simulink model "casihi"  (R2022b)
settings: Solver=VariableStepAuto  StartTime=0.0  StopTime=50  RelTol=1e-3
settings Model: Creator=10911  LastModifiedBy=acer
settings SolverCC: AlgebraicLoopSolver=TrustRegion
settings OptimizationCC: LifeSpan=inf
settings DebuggingCC: UnconnectedInputMsg=warning  UnconnectedOutputMsg=warning  UnconnectedLineMsg=warning  SFMachineParentedDataDiag=warning  ArithmeticOperatorsInVariantConditions=warning
settings ModelReferenceCC: EnableRefExpFcnMdlSchedulingChecks=on
settings SFSimCC: CustomCodeUndefinedFunction=UseInterfaceOnly
settings CodeAppCC: StateflowObjectComments=on

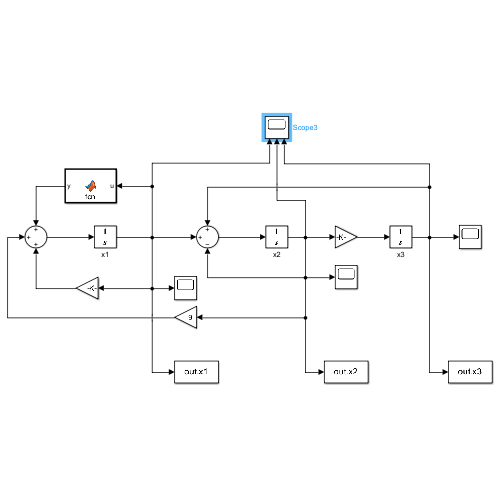
[thumbnail: Simulink's stored preview of the top-level diagram]
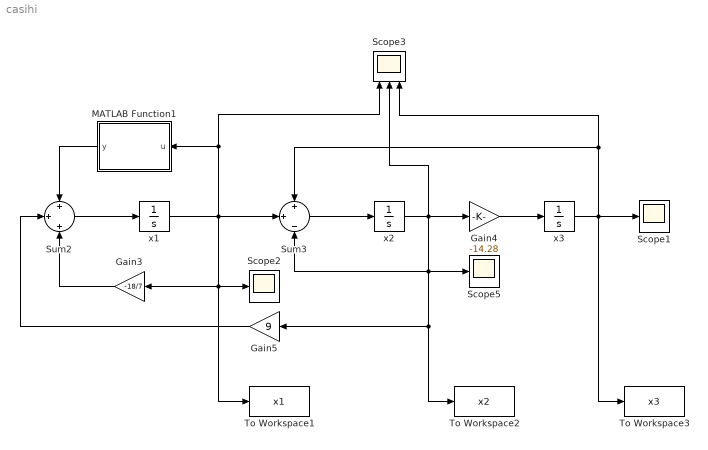
== system casihi ==
  Gain3 : Gain  Gain=-18/7
  Gain4 : Gain  Gain=-14.28
  Gain5 : Gain  Gain=9
  MATLAB Function1 : MATLAB Function  TreatAsAtomicUnit=on
  Scope1 : Scope
  Scope2 : Scope
  Scope3 : Scope  NumInputPorts=3
  Scope5 : Scope
  Sum2 : Sum  Inputs=+|+|+
  Sum3 : Sum  Inputs=+|+|-
  To Workspace1 : ToWorkspace  VariableName=x1  SaveFormat=Structure With Time  SampleTime=-1
  To Workspace2 : ToWorkspace  VariableName=x2  SaveFormat=Structure With Time  SampleTime=-1
  To Workspace3 : ToWorkspace  VariableName=x3  SaveFormat=Structure With Time  SampleTime=-1
  x1 : Integrator  InitialCondition=0.5
  x2 : Integrator  InitialCondition=0.5
  x3 : Integrator  InitialCondition=0.5
  wires:
  Sum2/1 -> x1/1
  x2/1 -> Scope3/2, Gain4/1, To Workspace2/1, Gain5/1, Sum3/3, Scope5/1
  x3/1 -> To Workspace3/1, Scope1/1, Sum3/1, Scope3/3
  Gain4/1 -> x3/1
  x1/1 -> Scope3/1, MATLAB Function1/1(u), Sum3/2, To Workspace1/1, Gain3/1, Scope2/1
  Sum3/1 -> x2/1
  Gain3/1 -> Sum2/3
  MATLAB Function1/1(y) -> Sum2/1
  Gain5/1 -> Sum2/2

== matlab function casihi/MATLAB Function1 ==
  data: u input; y output
function y = fcn(u)

y = 9*3/14*(abs(u+1)-abs(u-1));
